simulink model "os_pelny_regulacja"  (R2016b)
settings: Solver=FixedStepAuto  StartTime=0.0  StopTime=20  FixedStep=0.01  RelTol=1e-3  EnableMultiTasking=on
values from neighbouring files (symbols this model uses):
  A = [2  -4  -1; 4  -2  -1; -4  0  -1]    [matlab.mat]    (also in obserwator_stanu.m = [2 -4 -1)
  B = [0 0 -2]    [matlab.mat]    (also in obserwator_stanu.m = [0;0;-2])
  C = [1 0 0]    [matlab.mat]    (also in obserwator_stanu.m)
  D = 0    [matlab.mat]    (also in obserwator_stanu.m = [0])
  H = [11 -3.54166666667 12.9166666667]    [matlab.mat]    (also in obserwator_stanu.m = L')
  K = [4 -3.75 -1]    [matlab.mat]    (also in obserwator_stanu.m = acker(A,B,p))
  N = -3.25    [matlab.mat]    (also in obserwator_stanu.m = K*Nx+Nu)
undefined symbols (not defined in the file or in its folder): sigbuilder_block
settings Model: Creator=Pawel  LastModifiedBy=Admin
settings DataIOCC: LimitDataPoints=on
settings OptimizationCC: LifeSpan=inf
settings DebuggingCC: AllowSymbolicDim=off  SFUnexpectedBacktrackingDiag=warning  SFNoUnconditionalDefaultTransitionDiag=warning  SFExecutionAtInitializationDiag=none
settings ModelReferenceCC: PropagateSignalLabelsOutOfModel=off
settings GRTTargetCC: TargetLangStandard=C89/C90 (ANSI)
settings ConfigComp: CovMetricSettings=dw  CovHtmlReporting=on  CovSaveCumulativeToWorkspaceVar=on  CovSaveSingleToWorkspaceVar=on  CovExternalEMLEnable=off

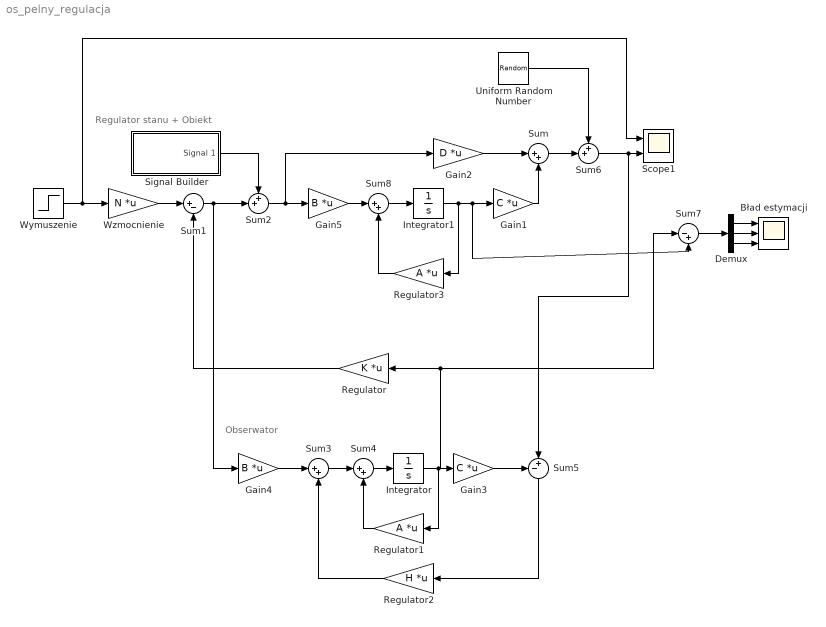
== system os_pelny_regulacja ==
  note: Obserwator
  note: Regulator stanu + Obiekt
  Bład estymacji : Scope  NumInputPorts=3
  Demux : Demux  Outputs=3
  Gain1 : Gain  Gain=C  Multiplication=Matrix(K*u)
  Gain2 : Gain  Gain=D  Multiplication=Matrix(K*u)
  Gain3 : Gain  Gain=C  Multiplication=Matrix(K*u)
  Gain4 : Gain  Gain=B  Multiplication=Matrix(K*u)
  Gain5 : Gain  Gain=B  Multiplication=Matrix(K*u)
  Integrator : Integrator
  Integrator1 : Integrator
  Regulator : Gain  Gain=K  Multiplication=Matrix(K*u)
  Regulator1 : Gain  Gain=A  Multiplication=Matrix(K*u)
  Regulator2 : Gain  Gain=H  Multiplication=Matrix(K*u)
  Regulator3 : Gain  Gain=A  Multiplication=Matrix(K*u)
  Scope1 : Scope  NumInputPorts=2
  Signal Builder : Subsystem  Tag=STV Subsys  LoadFcn=sigbuilder_block('load');  StartFcn=sigbuilder_block('start');  StopFcn=sigbuilder_block('stop');  ClipboardFcn=sigbuilder_block('clipboard');  mask(Sigbuilder block){tuvar=[0:10]}
      mask help: Simulink:masks:SigbuilderBlock_MD
      mask init:
      | if ~strcmp(get_param(bdroot(gcbh),'SimulationStatus'),'stopped') tuvar = sigbuilder_block('maskInit'); end
      settings: CopyFcn=sigbuilder_block('copy');  DeleteFcn=sigbuilder_block('delete');  ModelCloseFcn=sigbuilder_block('modelClose');  PreSaveFcn=sigbuilder_block('preSave');  PauseFcn=sigbuilder_block('pause');  ContinueFcn=sigbuilder_block('continue');  NameChangeFcn=sigbuilder_block('namechange');  OpenFcn=sigbuilder_block('open',[120.75 150 550.5 399.75 ]);  CloseFcn=sigbuilder_block('close');
      mask Display: plot(0, 0, 100, 100,[2, 2, 32, 32, 2], [68, 8, 8, 68, 68],[32, 2], [38, 38], [32, 19, 2],[53, 60, 44], [32, 17, 17, 2],[16, 16, 31, 31]);txt = getActiveGroup(gcbh);text(2, 100, txt,'verticalAlignment', 'top');
  Sum{,3..4,8} (4 alike) : Sum  Inputs=|++
  Sum1 : Sum  Inputs=|+-
  Sum2 : Sum  Inputs=++|
  Sum5 : Sum  Inputs=-+|
  Sum6 : Sum  Inputs=++|
  Sum7 : Sum  Inputs=|-+
  Uniform Random Number : UniformRandomNumber  Minimum=-0.005  Maximum=0.005  SampleTime=0.01
  Wymuszenie : Step  SampleTime=0
  Wzmocnienie : Gain  Gain=N  Multiplication=Matrix(K*u)
  wires:
  Wymuszenie/1 -> Wzmocnienie/1, Scope1/1
  Sum1/1 -> Sum2/2, Gain4/1
  Sum2/1 -> Gain5/1, Gain2/1
  Gain1/1 -> Sum/2
  Regulator/1 -> Sum1/2
  Integrator1/1 -> Regulator3/1, Gain1/1, Sum7/2
  Gain2/1 -> Sum/1
  Wzmocnienie/1 -> Sum1/1
  Sum3/1 -> Sum4/1
  Sum4/1 -> Integrator/1
  Integrator/1 -> Regulator/1, Sum7/1, Regulator1/1, Gain3/1
  Regulator1/1 -> Sum4/2
  Gain4/1 -> Sum3/1
  Gain3/1 -> Sum5/1
  Sum5/1 -> Regulator2/1
  Regulator2/1 -> Sum3/2
  Sum6/1 -> Sum5/2, Scope1/2
  Sum/1 -> Sum6/2
  Uniform Random Number/1 -> Sum6/1
  Gain5/1 -> Sum8/1
  Sum8/1 -> Integrator1/1
  Regulator3/1 -> Sum8/2
  Demux/1 -> Bład estymacji/1
  Sum7/1 -> Demux/1
  Demux/2 -> Bład estymacji/2
  Demux/3 -> Bład estymacji/3
  Signal Builder/1(Signal 1) -> Sum2/1

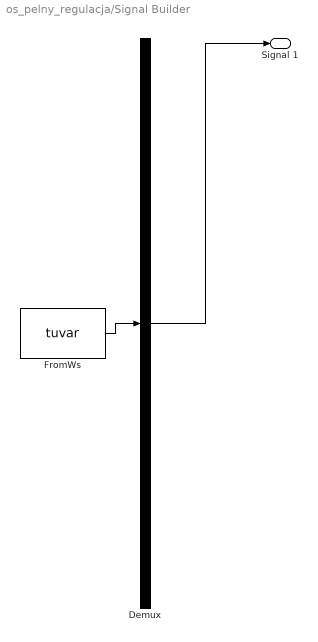
== system os_pelny_regulacja/Signal Builder ==
  Demux : Demux  Tag=STV Demux  Outputs=1
  FromWs : FromWorkspace  Tag=STV FromWs  VariableName=tuvar  SampleTime=0
      SigBuilderData=|
      | common.afterFinalStr = 'Extrapolate'
      | common.sampleTime = 0
      | dataSet.timeRange = [0 10]
      | dataSet.name = 'Group 1'
      | sbobj.Groups.Name = 'Group 1'
      | sbobj.Groups.Signals.Name = 'Signal 1'
      | sbobj.Groups.Signals.XData = [0 4 4 6 6 10]
      | sbobj.Groups.Signals.YData = [0 0 1 1 0 0]
  Signal 1 : Outport  Tag=STV Outport
  wires:
  Demux/1 -> Signal 1/1
  FromWs/1 -> Demux/1
